simulink model "Aircraft6dof"  (R2023b)
settings: Solver=ode4  StartTime=startTime  StopTime=stopTime  FixedStep=stepTime  RelTol=1e-3  EnableMultiTasking=on
values from neighbouring files (symbols this model uses):
  a0_s2 = 0    [SetupForTrimAndLin_Aircraft6dof.m]
  a0_s3 = 0    [SetupForTrimAndLin_Aircraft6dof.m]
  a0_s4 = 0.05    [SetupForTrimAndLin_Aircraft6dof.m]
  a0_s5 = 0.05    [SetupForTrimAndLin_Aircraft6dof.m]
  AR_s2 = b_s2 / c_s2    [SetupForTrimAndLin_Aircraft6dof.m]
  AR_s3 = b_s3 / c_s3    [SetupForTrimAndLin_Aircraft6dof.m]
  AR_s4 = (b_s4+b_s5) / c_s4    [SetupForTrimAndLin_Aircraft6dof.m]
  AR_s5 = (b_s4+b_s5) / c_s5    [SetupForTrimAndLin_Aircraft6dof.m]
  ARvecP1 = ARvecUIUCp1 * 30/pi * 2    [SetupForTrimAndLin_Aircraft6dof.m]
  c_s2 = componentMassesAndGeom(3,2)    [SetupForTrimAndLin_Aircraft6dof.m]
  c_s3 = componentMassesAndGeom(4,2)    [SetupForTrimAndLin_Aircraft6dof.m]
  c_s4 = componentMassesAndGeom(1,2)    [SetupForTrimAndLin_Aircraft6dof.m]
  c_s5 = componentMassesAndGeom(2,2)    [SetupForTrimAndLin_Aircraft6dof.m]
  CD0_s2 = 0.01    [SetupForTrimAndLin_Aircraft6dof.m]
  CD0_s3 = 0.01    [SetupForTrimAndLin_Aircraft6dof.m]
  CD0_s4 = 0.01    [SetupForTrimAndLin_Aircraft6dof.m]
  CD0_s5 = 0.01    [SetupForTrimAndLin_Aircraft6dof.m]
  CDa_s2 = 1    [SetupForTrimAndLin_Aircraft6dof.m]
  CDa_s3 = 1    [SetupForTrimAndLin_Aircraft6dof.m]
  CDa_s4 = 1    [SetupForTrimAndLin_Aircraft6dof.m]
  CDa_s5 = 1    [SetupForTrimAndLin_Aircraft6dof.m]
  CL0_s2 = 0    [SetupForTrimAndLin_Aircraft6dof.m]
  CL0_s3 = 0    [SetupForTrimAndLin_Aircraft6dof.m]
  CL0_s4 = 0.05    [SetupForTrimAndLin_Aircraft6dof.m]
  CL0_s5 = 0.05    [SetupForTrimAndLin_Aircraft6dof.m]
  CM0_s2 = 0    [SetupForTrimAndLin_Aircraft6dof.m]
  CM0_s3 = 0    [SetupForTrimAndLin_Aircraft6dof.m]
  CM0_s4 = -0.05    [SetupForTrimAndLin_Aircraft6dof.m]
  CM0_s5 = -0.05    [SetupForTrimAndLin_Aircraft6dof.m]
  CMa_s2 = 0    [SetupForTrimAndLin_Aircraft6dof.m]
  CMa_s3 = 0    [SetupForTrimAndLin_Aircraft6dof.m]
  CMa_s4 = 0    [SetupForTrimAndLin_Aircraft6dof.m]
  CMa_s5 = 0    [SetupForTrimAndLin_Aircraft6dof.m]
  CQvecP1 = CPvecP1    [SetupForTrimAndLin_Aircraft6dof.m]
  CTvecP1 = CTvecUIUCp1 * 2 * (1/(2*pi))^2 * (2^4)    [SetupForTrimAndLin_Aircraft6dof.m]
  dCL_du = 3    [SetupForTrimAndLin_Aircraft6dof.m]
  dE_0 = 0    [SetupForTrimAndLin_Aircraft6dof.m]
  dEL_0 = 0    [SetupForTrimAndLin_Aircraft6dof.m]
  DeMixMatrix = inv(MixMatrix)    [SetupForTrimAndLin_Aircraft6dof.m]
  dER_0 = 0    [SetupForTrimAndLin_Aircraft6dof.m]
  dR_0 = 0    [SetupForTrimAndLin_Aircraft6dof.m]
  e_s2 = 0.8    [SetupForTrimAndLin_Aircraft6dof.m]
  e_s3 = 0.8    [SetupForTrimAndLin_Aircraft6dof.m]
  e_s4 = 0.9    [SetupForTrimAndLin_Aircraft6dof.m]
  e_s5 = 0.9    [SetupForTrimAndLin_Aircraft6dof.m]
  elevator_vector = [0  0  0.1    0.1   -0.1    -0.1  0       0  ]    [SetupAndRun_Aircraft6dof.m]
  g_E_N = [0; 0; 9.81]*1    [SetupAndRun_Aircraft6dof.m]    (also in SetupForTrimAndLin_Aircraft6dof.m = [0; 0; 9.81])
  i_s2 = -0.1    [SetupForTrimAndLin_Aircraft6dof.m]
  i_s3 = 0    [SetupForTrimAndLin_Aircraft6dof.m]
  i_s4 = 0.0    (= 0)    [SetupForTrimAndLin_Aircraft6dof.m]
  i_s5 = 0.0    (= 0)    [SetupForTrimAndLin_Aircraft6dof.m]
  InitAtt = InitAtt_deg * deg2rad    [SetupAndRun_Aircraft6dof.m]    (also in SetupForTrimAndLin_Aircraft6dof.m)
  InitPos = InitPos_deg .* [deg2rad; deg2rad; 1]    [SetupAndRun_Aircraft6dof.m]    (also in SetupForTrimAndLin_Aircraft6dof.m)
  InitRates = Rates_Trim    [SetupAndRun_Aircraft6dof.m]    (also in SetupForTrimAndLin_Aircraft6dof.m = [0; 0; 0])
  InitVel = Vel_B_BA_Trim    [SetupAndRun_Aircraft6dof.m]    (also in SetupForTrimAndLin_Aircraft6dof.m = [15; 0; 0])
  Io_motor = 1.6    [SetupForTrimAndLin_Aircraft6dof.m]
  J = zeros(3,3)    [DefineAircraftGeometry.m]    (also in InitializeModel.m = ASW.RotationalInertiaMatrix; SetupAndRun_Aircraft6dof.m = [0.049 0 -0.0004; 0 0.022 0; -0.0004 0 0.071]; SetupForTrimAndLin_Aircraft6dof.m)
  Ki_motor = 0.009549    [SetupForTrimAndLin_Aircraft6dof.m]
  m = sum(obj.componentMassesAndGeom(:,1))    [DefineAircraftGeometry.m]    (also in SetupForTrimAndLin_Aircraft6dof.m = sum(componentMassesAndGeom(:,1)))
  MixMatrix = [-1 1 0 0 ... (first row only)    [SetupForTrimAndLin_Aircraft6dof.m]
  n_p1 = [1; 0; 0]    [SetupForTrimAndLin_Aircraft6dof.m]
  n_s2 = [0; 0; -1]    [SetupForTrimAndLin_Aircraft6dof.m]
  n_s3 = [0; 1; 0]    [SetupForTrimAndLin_Aircraft6dof.m]
  n_s4 = [0; sin(0*pi/180);  -cos(0*pi/180)]    [SetupForTrimAndLin_Aircraft6dof.m]
  n_s5 = [0; sin(0*pi/180);  -cos(0*pi/180)]    [SetupForTrimAndLin_Aircraft6dof.m]
  nCellsSeries = 6    [SetupForTrimAndLin_Aircraft6dof.m]
  om_motor_init = 0    [SetupForTrimAndLin_Aircraft6dof.m]
  R_p1 = componentMassesAndGeom(11,3)/2    [SetupForTrimAndLin_Aircraft6dof.m]
  Rearth = 6371000    [SetupForTrimAndLin_Aircraft6dof.m]
  Rmotor = 0.4    [SetupForTrimAndLin_Aircraft6dof.m]
  rudder_vector = [0  0  -0.1   -0.1 0      0     0.1     0.1   0       0  ]    [SetupAndRun_Aircraft6dof.m]
  S_s2 = c_s2 * b_s2    [SetupForTrimAndLin_Aircraft6dof.m]
  S_s3 = c_s3 * b_s3    [SetupForTrimAndLin_Aircraft6dof.m]
  S_s4 = c_s4 * b_s4    [SetupForTrimAndLin_Aircraft6dof.m]
  S_s5 = c_s5 * b_s5    [SetupForTrimAndLin_Aircraft6dof.m]
  S_u_s2 = c_u_s2*b_s2    [SetupForTrimAndLin_Aircraft6dof.m]
  S_u_s3 = c_u_s3*b_s3    [SetupForTrimAndLin_Aircraft6dof.m]
  S_u_s4 = c_u_s4*b_s4    [SetupForTrimAndLin_Aircraft6dof.m]
  S_u_s5 = c_u_s5*b_s5    [SetupForTrimAndLin_Aircraft6dof.m]
  tauE = 0.1    [SetupForTrimAndLin_Aircraft6dof.m]
  tauEL = 0.1    [SetupForTrimAndLin_Aircraft6dof.m]
  tauER = 0.1    [SetupForTrimAndLin_Aircraft6dof.m]
  tauR = 0.1    [SetupForTrimAndLin_Aircraft6dof.m]
  time_vector_elevator = [0  10 10.001 100   100.001 200   200.001 10000]    [SetupAndRun_Aircraft6dof.m]
  time_vector_rudder = [0  10 10.001 70   70.001 200   200.001 300   300.001 10000]    [SetupAndRun_Aircraft6dof.m]
  v_N_AE = [0; 0; 0]    [SetupAndRun_Aircraft6dof.m]    (also in SetupForTrimAndLin_Aircraft6dof.m)
  VcellMax = 4.2    [SetupForTrimAndLin_Aircraft6dof.m]
  Vel_W_Trim = [norm(Vel_B_BA_Trim); atan2(Vel_B_BA_Trim(3),Vel_B_BA_Trim(1)); asin(Vel_B_BA_Trim(2)/norm(Vel_B_BA_Trim)) ]    [TrimAndLinearize_ATT_wInputs_Aircraft6dof.m]
  x_cm = sum(obj.componentMassesAndGeom(:,1) .* obj.componentMassesAndGeom(:,5:7)) / m    [DefineAircraftGeometry.m]    (also in SetupForTrimAndLin_Aircraft6dof.m = x_cm')
  x_p1 = componentMassesAndGeom(11,5:7)'    [SetupForTrimAndLin_Aircraft6dof.m]
  x_s2 = [componentMassesAndGeom(3,5) + (1/4)*componentMassesAndGeom(3,2); componentMassesAndGeom(3,6);componentMassesAndGeom(3,7)]    [SetupForTrimAndLin_Aircraft6dof.m]
  x_s3 = [componentMassesAndGeom(4,5) + (1/4)*componentMassesAndGeom(4,2); componentMassesAndGeom(4,6);componentMassesAndGeom(4,7)]    [SetupForTrimAndLin_Aircraft6dof.m]
  x_s4 = [componentMassesAndGeom(1,5) + (1/4)*componentMassesAndGeom(1,2); componentMassesAndGeom(1,6);componentMassesAndGeom(1,7)]    [SetupForTrimAndLin_Aircraft6dof.m]
  x_s5 = [componentMassesAndGeom(2,5) + (1/4)*componentMassesAndGeom(2,2); componentMassesAndGeom(2,6);componentMassesAndGeom(2,7)]    [SetupForTrimAndLin_Aircraft6dof.m]
undefined symbols (not defined in the file or in its folder): InitQuat, J_int, K_decouple, K_lqr, n_int, reg_lqg, X_trim, Y_trim
libraries: vrlib x8, simulink x7, aerolibfltsims x1
(part 1 of 3)
settings Model: Creator=McArthur  LastModifiedBy=prafulsigdel
settings SolverCC: AlgebraicLoopSolver=TrustRegion
settings DataIOCC: LimitDataPoints=on  SaveFormat=StructureWithTime  ReturnWorkspaceOutputs=off
settings OptimizationCC: LifeSpan=inf
settings DebuggingCC: UnconnectedInputMsg=warning  UnconnectedOutputMsg=warning  UnconnectedLineMsg=warning  SFUnexpectedBacktrackingDiag=warning  SFNoUnconditionalDefaultTransitionDiag=warning  SFExecutionAtInitializationDiag=none  ArithmeticOperatorsInVariantConditions=warning
settings HardwareCC: ProdBitPerSizeT=32  ProdBitPerPtrDiffT=32  ProdWordSize=32  ProdHWDeviceType=Specified
settings ModelReferenceCC: EnableRefExpFcnMdlSchedulingChecks=on  PropagateSignalLabelsOutOfModel=off
settings SFSimCC: SimUseLocalCustomCode=off  CustomCodeUndefinedFunction=UseInterfaceOnly
settings RTWCC: RTWUseLocalCustomCode=off
settings CodeAppCC: StateflowObjectComments=on
settings GRTTargetCC: TargetLangStandard=C89/C90 (ANSI)
settings ConfigComp: CovMetricSettings=dw  CovSaveCumulativeToWorkspaceVar=on  CovSaveSingleToWorkspaceVar=on  CovExternalEMLEnable=off

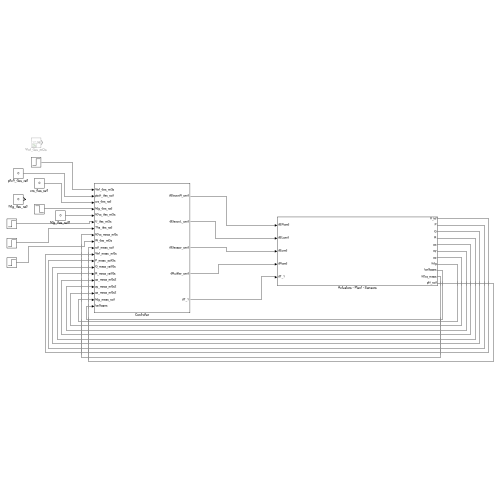
[thumbnail: Simulink's stored preview of the top-level diagram]
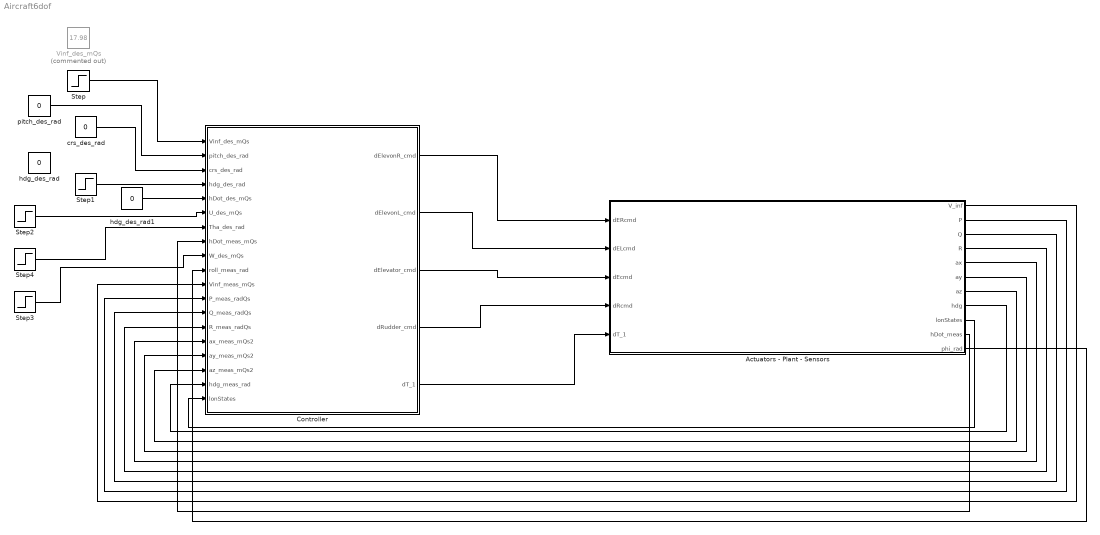
== system Aircraft6dof ==
  Actuators - Plant - Sensors : Subsystem
  Controller : Subsystem
  Step : Step  Time=9  Before=Vel_W_Trim(1)  After=Vel_W_Trim(1)+3  SampleTime=0
  Step1 : Step  Time=21  After=-170*pi/180  SampleTime=0
  Step2 : Step  Time=9  Before=X_trim(4)  After=X_trim(4)+3  SampleTime=0
  Step3 : Step  Time=9  Before=X_trim(6)  After=X_trim(6)  SampleTime=0
  Step4 : Step  Time=9  Before=X_trim(2)  After=X_trim(2)  SampleTime=0
  Vinf_des_mQs : Constant  Commented=on  Value=17.98
  crs_des_rad : Constant  Value=0
  hdg_des_rad : Constant  Value=0
  hdg_des_rad1 : Constant  Value=0
  pitch_des_rad : Constant  Value=0
  wires:
  Actuators - Plant - Sensors/1(V_inf) -> Controller/11(Vinf_meas_mQs)
  Actuators - Plant - Sensors/8(hdg) -> Controller/18(hdg_meas_rad)
  Actuators - Plant - Sensors/7(az) -> Controller/17(az_meas_mQs2)
  Actuators - Plant - Sensors/6(ay) -> Controller/16(ay_meas_mQs2)
  Actuators - Plant - Sensors/5(ax) -> Controller/15(ax_meas_mQs2)
  Actuators - Plant - Sensors/4(R) -> Controller/14(R_meas_radQs)
  Actuators - Plant - Sensors/3(Q) -> Controller/13(Q_meas_radQs)
  Actuators - Plant - Sensors/2(P) -> Controller/12(P_meas_radQs)
  Step/1 -> Controller/1(Vinf_des_mQs)
  pitch_des_rad/1 -> Controller/2(pitch_des_rad)
  crs_des_rad/1 -> Controller/3(crs_des_rad)
  Step1/1 -> Controller/4(hdg_des_rad)
  Controller/2(dElevonL_cmd) -> Actuators - Plant - Sensors/2(dELcmd)
  Controller/1(dElevonR_cmd) -> Actuators - Plant - Sensors/1(dERcmd)
  Controller/3(dElevator_cmd) -> Actuators - Plant - Sensors/3(dEcmd)
  Controller/4(dRudder_cmd) -> Actuators - Plant - Sensors/4(dRcmd)
  Actuators - Plant - Sensors/9(lonStates) -> Controller/19(lonStates)
  Step3/1 -> Controller/9(W_des_mQs)
  Step4/1 -> Controller/7(Tha_des_rad)
  Step2/1 -> Controller/6(U_des_mQs)
  Controller/5(dT_1) -> Actuators - Plant - Sensors/5(dT_1)
  hdg_des_rad1/1 -> Controller/5(hDot_des_mQs)
  Actuators - Plant - Sensors/10(hDot_meas) -> Controller/8(hDot_meas_mQs)
  Actuators - Plant - Sensors/11(phi_rad) -> Controller/10(roll_meas_rad)

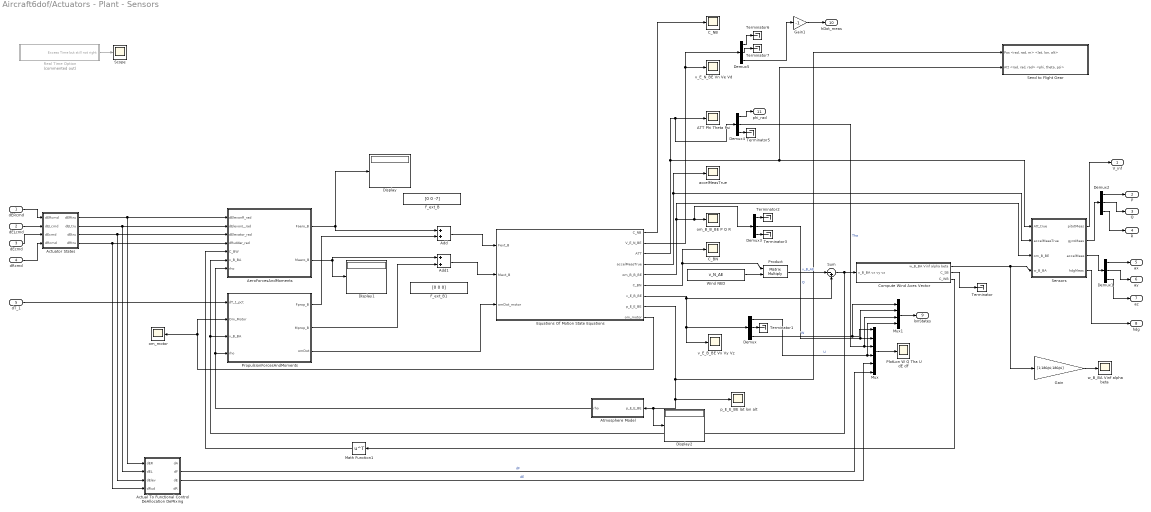
== system Aircraft6dof/Actuators - Plant - Sensors ==
  dERcmd : Inport
  dELcmd : Inport  Port=2
  dEcmd : Inport  Port=3
  dRcmd : Inport  Port=4
  dT_1 : Inport  Port=5
  ATT Phi Theta Psi : Scope
  Actual To Functional Control DeAllocation DeMixing : Subsystem
  Actuator States : Subsystem
  Add : Sum
  Add1 : Sum
  AeroForcesAndMoments : Subsystem
  Atmosphere Model : Subsystem
  C_BN : Scope
  C_NB : Scope
  Compute Wind Axes Vector : Subsystem
  Demux{,1..5} (6 alike) : Demux  Outputs=3
  Display : Display
  Display1 : Display
  Display2 : Display
  Equations Of Motion State Equations : Subsystem
  F_ext_B : Constant  Value=[0 0 -7]
  F_ext_B1 : Constant  Value=[0 0 0]
  Gain : Gain  Gain=[1;180/pi;180/pi]
  Gain1 : Gain  Gain=-1
  Math Function1 : Math  Operator=transpose  SignedPower=on
  Mux : Mux  Inputs=6
  Mux1 : Mux
  PlotLon W Q Tha U dE dF : Scope
  Product : Product  Multiplication=Matrix(*)
  PropulsionForcesAndMoments : Subsystem
  Real Time Option : Subsystem  Commented=on
  Scope : Scope
  Send to Flight Gear : Subsystem
  Sensors : Subsystem
  Sum : Sum  Inputs=|-+
  Terminator{,1..3,5..7} (7 alike) : Terminator
  Wind NED : Constant  Value=v_N_AE
  accelMeasTrue : Scope
  om_B_B_BE P Q R : Scope
  om_motor : Scope
  p_E_E_BE lat lon alt : Scope
  v_E_B_BE Vx Vy Vz : Scope
  v_E_N_BE Vn Ve Vd : Scope
  w_B_BA Vinf alpha beta : Scope
  V_inf : Outport  VectorParamsAs1DForOutWhenUnconnected=off
  P : Outport  Port=2  VectorParamsAs1DForOutWhenUnconnected=off
  Q : Outport  Port=3  VectorParamsAs1DForOutWhenUnconnected=off
  R : Outport  Port=4  VectorParamsAs1DForOutWhenUnconnected=off
  ax : Outport  Port=5  VectorParamsAs1DForOutWhenUnconnected=off
  ay : Outport  Port=6  VectorParamsAs1DForOutWhenUnconnected=off
  az : Outport  Port=7  VectorParamsAs1DForOutWhenUnconnected=off
  hdg : Outport  Port=8  VectorParamsAs1DForOutWhenUnconnected=off
  lonStates : Outport  Port=9  VectorParamsAs1DForOutWhenUnconnected=off
  hDot_meas : Outport  Port=10  VectorParamsAs1DForOutWhenUnconnected=off
  phi_rad : Outport  Port=11  VectorParamsAs1DForOutWhenUnconnected=off
  wires:
  Real Time Option/1(Excess Time but still not right) -> Scope/1
  AeroForcesAndMoments/2(Maero_B) -> Add1/1, Display1/1
  PropulsionForcesAndMoments/3(omDot) -> Equations Of Motion State Equations/3(omDot_motor)
  AeroForcesAndMoments/1(Faero_B) -> Add/1, Display/1
  Equations Of Motion State Equations/8(p_E_E_BE) -> Send to Flight Gear/1("Pos <rad, rad, m> <lat, lon, alt>"), Display2/1, Atmosphere Model/1(p_E_E_BE), p_E_E_BE lat lon alt/1
  Equations Of Motion State Equations/2(V_E_N_BE) -> Demux5/1, v_E_N_BE Vn Ve Vd/1
  Equations Of Motion State Equations/1(C_NB) -> C_NB/1
  Sum/1 -> PropulsionForcesAndMoments/3(v_B_BA), AeroForcesAndMoments/6(v_B_BA), Compute Wind Axes Vector/1(v_B_BA vx vy vz)
  Compute Wind Axes Vector/3(C_WB) -> Math Function1/1
  Math Function1/1 -> AeroForcesAndMoments/5(C_BW)
  Equations Of Motion State Equations/5(om_B_B_BE) -> Sensors/3(om_B_BE), Demux3/1, om_B_B_BE P Q R/1
  Equations Of Motion State Equations/6(C_BN) -> C_BN/1, Product/1
  Demux2/2 -> Q/1
  Demux2/3 -> R/1
  Demux2/1 -> P/1
  Product/1 -> Sum/1  "v_B_AE"
  Gain/1 -> w_B_BA Vinf alpha beta/1
  Atmosphere Model/1(rho) -> PropulsionForcesAndMoments/4(rho), AeroForcesAndMoments/7(rho)
  Compute Wind Axes Vector/1(w_B_BA Vinf alpha beta) -> Gain/1, Sensors/4(w_B_BA)
  Compute Wind Axes Vector/2(C_SB) -> Terminator/1
  Equations Of Motion State Equations/7(v_E_B_BE) -> Sum/2, v_E_B_BE Vx Vy Vz/1, Demux/1
  Sensors/1(pitotMeas) -> V_inf/1
  Sensors/2(gyroMeas) -> Demux2/1
  Equations Of Motion State Equations/4(accelMeasTrue) -> Sensors/2(accelMeasTrue), accelMeasTrue/1
  Wind NED/1 -> Product/2
  Demux1/1 -> ax/1
  Demux1/2 -> ay/1
  Demux1/3 -> az/1
  Sensors/3(accelMeas) -> Demux1/1
  Sensors/4(hdgMeas) -> hdg/1
  Actuator States/4(dRtru) -> Actual To Functional Control DeAllocation DeMixing/4(dRud), AeroForcesAndMoments/4(dRudder_rad)
  Actuator States/3(dEtru) -> Actual To Functional Control DeAllocation DeMixing/3(dElev), AeroForcesAndMoments/3(dElevator_rad)
  Actuator States/2(dELtru) -> Actual To Functional Control DeAllocation DeMixing/2(dEL), AeroForcesAndMoments/2(dElevonL_rad)
  Actuator States/1(dERtru) -> Actual To Functional Control DeAllocation DeMixing/1(dER), AeroForcesAndMoments/1(dElevonR_rad)
  dERcmd/1 -> Actuator States/1(dERcmd)
  dELcmd/1 -> Actuator States/2(dELcmd)
  dEcmd/1 -> Actuator States/3(dEcmd)
  dRcmd/1 -> Actuator States/4(dRcmd)
  Mux/1 -> PlotLon W Q Tha U dE dF/1
  Demux/3 -> Mux1/1, Mux/1  "W"
  Demux/1 -> Mux1/4, Mux/4  "U"
  Demux/2 -> Terminator1/1
  Demux3/2 -> Mux1/2, Mux/2  "Q"
  Demux3/1 -> Terminator2/1
  Demux3/3 -> Terminator3/1
  Equations Of Motion State Equations/3(ATT) -> Demux4/1, ATT Phi Theta Psi/1, Send to Flight Gear/2("Att <rad, rad, rad> <phi, theta, psi>"), Sensors/1(Att_true)
  Demux4/2 -> Mux1/3, Mux/3  "Tha"
  Demux4/1 -> phi_rad/1
  Demux4/3 -> Terminator5/1
  Actual To Functional Control DeAllocation DeMixing/3(dE) -> Mux/5  "dE"
  Actual To Functional Control DeAllocation DeMixing/2(dF) -> Mux/6  "dF"
  Mux1/1 -> lonStates/1
  Add/1 -> Equations Of Motion State Equations/1(Fext_B)
  Add1/1 -> Equations Of Motion State Equations/2(Mext_B)
  dT_1/1 -> PropulsionForcesAndMoments/1(dT_1_pct)
  Equations Of Motion State Equations/9(om_motor) -> PropulsionForcesAndMoments/2(Om_Motor), om_motor/1
  PropulsionForcesAndMoments/1(Fprop_B) -> Add/2
  PropulsionForcesAndMoments/2(Mprop_B) -> Add1/2
  Demux5/3 -> Gain1/1
  Gain1/1 -> hDot_meas/1
  Demux5/1 -> Terminator6/1
  Demux5/2 -> Terminator7/1

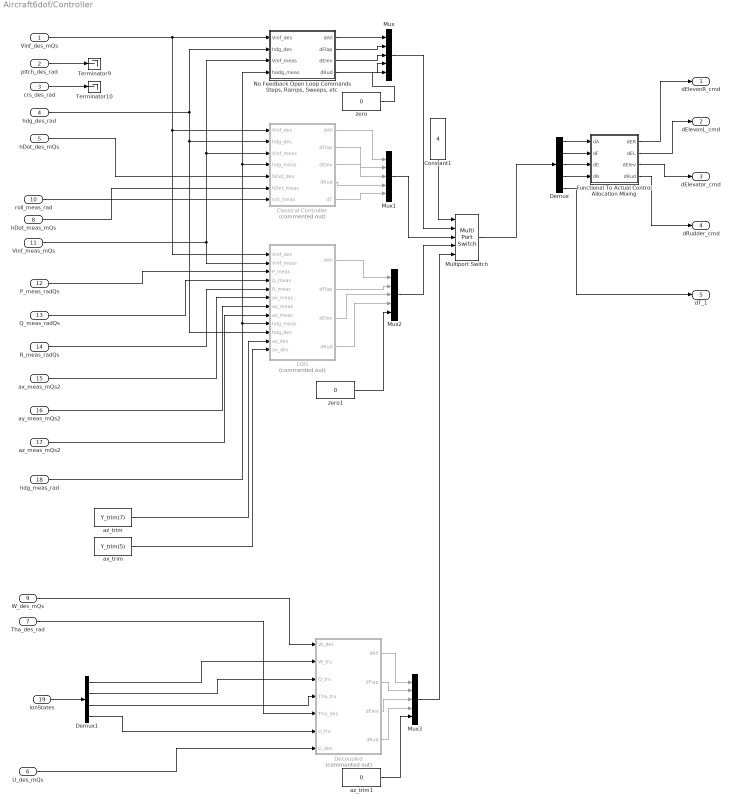
== system Aircraft6dof/Controller ==
  Vinf_des_mQs : Inport
  pitch_des_rad : Inport  Port=2
  crs_des_rad : Inport  Port=3
  hdg_des_rad : Inport  Port=4
  hDot_des_mQs : Inport  Port=5
  U_des_mQs : Inport  Port=6
  Tha_des_rad : Inport  Port=7
  hDot_meas_mQs : Inport  Port=8
  W_des_mQs : Inport  Port=9
  roll_meas_rad : Inport  Port=10
  Vinf_meas_mQs : Inport  Port=11
  P_meas_radQs : Inport  Port=12
  Q_meas_radQs : Inport  Port=13
  R_meas_radQs : Inport  Port=14
  ax_meas_mQs2 : Inport  Port=15
  ay_meas_mQs2 : Inport  Port=16
  az_meas_mQs2 : Inport  Port=17
  hdg_meas_rad : Inport  Port=18
  lonStates : Inport  Port=19
  Classical Controller : Subsystem  Commented=on
  Constant1 : Constant  Value=4
  Decoupled : Subsystem  Commented=on
  Demux : Demux  Outputs=5
  Demux1 : Demux
  Functional To Actual Control Allocation Mixing : Subsystem
  LQG : Subsystem  Commented=on
  Multiport Switch : MultiPortSwitch  Inputs=4  SaturateOnIntegerOverflow=off  InputSameDT=off
  Mux{,1..3} (4 alike) : Mux  Inputs=5
  "No Feedback Open Loop Commands Steps, Ramps, Sweeps, etc" : Subsystem
  Terminator10 : Terminator
  Terminator9 : Terminator
  ax_trim : Constant  Value=Y_trim(5)
  az_trim : Constant  Value=Y_trim(7)
  az_trim1 : Constant  Value=0
  zero : Constant  Value=0
  zero1 : Constant  Value=0
  dElevonR_cmd : Outport  VectorParamsAs1DForOutWhenUnconnected=off
  dElevonL_cmd : Outport  Port=2  VectorParamsAs1DForOutWhenUnconnected=off
  dElevator_cmd : Outport  Port=3  VectorParamsAs1DForOutWhenUnconnected=off
  dRudder_cmd : Outport  Port=4  VectorParamsAs1DForOutWhenUnconnected=off
  dT_1 : Outport  Port=5  VectorParamsAs1DForOutWhenUnconnected=off
  wires:
  P_meas_radQs/1 -> LQG/3(P_meas)
  Q_meas_radQs/1 -> LQG/4(Q_meas)
  ay_meas_mQs2/1 -> LQG/7(ay_meas)
  ax_meas_mQs2/1 -> LQG/6(ax_meas)
  R_meas_radQs/1 -> LQG/5(R_meas)
  az_meas_mQs2/1 -> LQG/8(az_meas)
  crs_des_rad/1 -> Terminator10/1
  pitch_des_rad/1 -> Terminator9/1
  Functional To Actual Control Allocation Mixing/1(dER) -> dElevonR_cmd/1
  Functional To Actual Control Allocation Mixing/2(dEL) -> dElevonL_cmd/1
  Functional To Actual Control Allocation Mixing/3(dElev) -> dElevator_cmd/1
  Functional To Actual Control Allocation Mixing/4(dRud) -> dRudder_cmd/1
  hdg_des_rad/1 -> LQG/10(hdg_des), Classical Controller/2(hdg_des), "No Feedback Open Loop Commands Steps, Ramps, Sweeps, etc"/2(hdg_des)
  Vinf_meas_mQs/1 -> LQG/2(Vinf_meas), "No Feedback Open Loop Commands Steps, Ramps, Sweeps, etc"/3(Vinf_meas), Classical Controller/3(Vinf_meas)
  hdg_meas_rad/1 -> Classical Controller/4(hdg_meas), "No Feedback Open Loop Commands Steps, Ramps, Sweeps, etc"/4(hadg_meas), LQG/9(hdg_meas)
  "No Feedback Open Loop Commands Steps, Ramps, Sweeps, etc"/1(dAil) -> Mux/1
  "No Feedback Open Loop Commands Steps, Ramps, Sweeps, etc"/2(dFlap) -> Mux/2
  "No Feedback Open Loop Commands Steps, Ramps, Sweeps, etc"/3(dElev) -> Mux/3
  "No Feedback Open Loop Commands Steps, Ramps, Sweeps, etc"/4(dRud) -> Mux/4
  Mux/1 -> Multiport Switch/2
  Constant1/1 -> Multiport Switch/1
  Classical Controller/1(dAil) -> Mux1/1
  Classical Controller/4(dRud) -> Mux1/4
  Classical Controller/3(dElev) -> Mux1/3
  Classical Controller/2(dFlap) -> Mux1/2
  Mux1/1 -> Multiport Switch/3
  Demux/3 -> Functional To Actual Control Allocation Mixing/3(dE)
  Demux/2 -> Functional To Actual Control Allocation Mixing/2(dF)
  Demux/1 -> Functional To Actual Control Allocation Mixing/1(dA)
  Demux/4 -> Functional To Actual Control Allocation Mixing/4(dR)
  Multiport Switch/1 -> Demux/1
  LQG/1(dAil) -> Mux2/1
  LQG/4(dRud) -> Mux2/4
  LQG/3(dElev) -> Mux2/3
  LQG/2(dFlap) -> Mux2/2
  Mux2/1 -> Multiport Switch/4
  Vinf_des_mQs/1 -> "No Feedback Open Loop Commands Steps, Ramps, Sweeps, etc"/1(Vinf_des), LQG/1(Vinf_des), Classical Controller/1(Vinf_des)
  az_trim/1 -> LQG/11(az_des)
  ax_trim/1 -> LQG/12(ax_des)
  Decoupled/1(dAil) -> Mux3/1
  Decoupled/2(dFlap) -> Mux3/2
  Decoupled/3(dElev) -> Mux3/3
  Decoupled/4(dRud) -> Mux3/4
  Mux3/1 -> Multiport Switch/5
  lonStates/1 -> Demux1/1
  Demux1/1 -> Decoupled/2(W_tru)
  Demux1/2 -> Decoupled/3(Q_tru)
  Demux1/3 -> Decoupled/4(Tha_tru)
  Demux1/4 -> Decoupled/6(U_tru)
  W_des_mQs/1 -> Decoupled/1(W_des)
  Tha_des_rad/1 -> Decoupled/5(Tha_des)
  U_des_mQs/1 -> Decoupled/7(U_des)
  Demux/5 -> dT_1/1
  hDot_des_mQs/1 -> Classical Controller/5(hDot_des)
  hDot_meas_mQs/1 -> Classical Controller/6(hDot_meas)
  roll_meas_rad/1 -> Classical Controller/7(roll_meas)
  Classical Controller/5(dT) -> Mux1/5
  zero/1 -> Mux/5
  zero1/1 -> Mux2/5
  az_trim1/1 -> Mux3/5

== system Aircraft6dof/Actuators - Plant - Sensors/Actual To Functional Control DeAllocation DeMixing ==
  dER : Inport
  dEL : Inport  Port=2
  dElev : Inport  Port=3
  dRud : Inport  Port=4
  Constant1 : Constant  Value=DeMixMatrix
  Demux : Demux
  Mux : Mux
  Product1 : Product  Multiplication=Matrix(*)
  dA : Outport  VectorParamsAs1DForOutWhenUnconnected=off
  dF : Outport  Port=2  VectorParamsAs1DForOutWhenUnconnected=off
  dE : Outport  Port=3  VectorParamsAs1DForOutWhenUnconnected=off
  dR : Outport  Port=4  VectorParamsAs1DForOutWhenUnconnected=off
  wires:
  dER/1 -> Mux/1
  dEL/1 -> Mux/2
  dElev/1 -> Mux/3
  dRud/1 -> Mux/4
  Demux/2 -> dF/1
  Constant1/1 -> Product1/1
  Mux/1 -> Product1/2
  Demux/1 -> dA/1
  Demux/4 -> dR/1
  Demux/3 -> dE/1
  Product1/1 -> Demux/1

== system Aircraft6dof/Actuators - Plant - Sensors/Actuator States ==
  dERcmd : Inport
  dELcmd : Inport  Port=2
  dEcmd : Inport  Port=3
  dRcmd : Inport  Port=4
  Constant : Constant  Value=dER_0
  Constant1 : Constant  Value=dEL_0
  Constant2 : Constant  Value=dE_0
  Constant3 : Constant  Value=dR_0
  Gain : Gain  Gain=1/tauER
  Gain1 : Gain  Gain=1/tauEL
  Gain2 : Gain  Gain=1/tauE
  Gain3 : Gain  Gain=1/tauR
  Sum{,1..3} (4 alike) : Sum  Inputs=|+-
  dE : Integrator  InitialConditionSource=external
  dEL : Integrator  InitialConditionSource=external
  dER : Integrator  InitialConditionSource=external
  dR : Integrator  InitialConditionSource=external
  dERtru : Outport  VectorParamsAs1DForOutWhenUnconnected=off
  dELtru : Outport  Port=2  VectorParamsAs1DForOutWhenUnconnected=off
  dEtru : Outport  Port=3  VectorParamsAs1DForOutWhenUnconnected=off
  dRtru : Outport  Port=4  VectorParamsAs1DForOutWhenUnconnected=off
  wires:
  dER/1 -> Sum/2, dERtru/1
  dERcmd/1 -> Sum/1
  Gain/1 -> dER/1
  Sum/1 -> Gain/1
  Constant/1 -> dER/2
  dEL/1 -> Sum1/2, dELtru/1
  dELcmd/1 -> Sum1/1
  Gain1/1 -> dEL/1
  Sum1/1 -> Gain1/1
  Constant1/1 -> dEL/2
  dE/1 -> Sum2/2, dEtru/1
  dEcmd/1 -> Sum2/1
  Gain2/1 -> dE/1
  Sum2/1 -> Gain2/1
  Constant2/1 -> dE/2
  dR/1 -> Sum3/2, dRtru/1
  dRcmd/1 -> Sum3/1
  Gain3/1 -> dR/1
  Sum3/1 -> Gain3/1
  Constant3/1 -> dR/2

== system Aircraft6dof/Actuators - Plant - Sensors/AeroForcesAndMoments ==
  dElevonR_rad : Inport
  dElevonL_rad : Inport  Port=2
  dElevator_rad : Inport  Port=3
  dRudder_rad : Inport  Port=4
  C_BW : Inport  Port=5
  v_B_BA : Inport  Port=6
  rho : Inport  Port=7
  Add : Sum  Inputs=++++
  Add1 : Sum  Inputs=++++
  Display1 : Display
  Display3 : Display
  Surface2 : Subsystem
  Surface3 : Subsystem
  Surface4 : Subsystem
  Surface5 : Subsystem
  Faero_B : Outport  VectorParamsAs1DForOutWhenUnconnected=off
  Maero_B : Outport  Port=2  VectorParamsAs1DForOutWhenUnconnected=off
  wires:
  C_BW/1 -> Surface2/1(C_BW), Surface3/1(C_BW), Surface5/1(C_BW), Surface4/1(C_BW)
  v_B_BA/1 -> Surface3/2(v_B_BA), Surface2/2(v_B_BA), Surface5/2(v_B_BA), Surface4/2(v_B_BA)
  rho/1 -> Surface3/3(rho), Surface2/3(rho), Surface5/3(rho), Surface4/3(rho)
  Surface4/1(Fs4_B) -> Add/1
  Surface5/1(Fs5_B) -> Add/2
  Surface4/2(Ms4_B) -> Add1/1
  Surface5/2(Ms5_B) -> Add1/2
  Surface2/1(Fs2_B) -> Add/3
  Surface2/2(Ms2_B) -> Add1/3
  Add1/1 -> Display1/1, Maero_B/1
  Add/1 -> Display3/1, Faero_B/1
  Surface3/1(Fs2_B) -> Add/4
  Surface3/2(Ms2_B) -> Add1/4
  dElevonR_rad/1 -> Surface4/4(u_s#_rad)
  dElevonL_rad/1 -> Surface5/4(u_s#_rad)
  dElevator_rad/1 -> Surface2/4(u_s#_rad)
  dRudder_rad/1 -> Surface3/4(u_s#_rad)

== system Aircraft6dof/Actuators - Plant - Sensors/Atmosphere Model ==
  p_E_E_BE : Inport
  Compare To Constant : simulink/Logic and Bit Operations/Compare To Constant  relop=<=  const=11000  OutDataTypeStr=boolean
  Demux : Demux  Outputs=3
  Enhance Me Please! : Constant  Value=0
  Standard Atmosphere - Troposphere : MATLAB Function  TreatAsAtomicUnit=on
  Switch : Switch  Criteria=u2 ~= 0  Threshold=11000  SaturateOnIntegerOverflow=off  InputSameDT=off
  Terminator : Terminator
  Terminator1 : Terminator
  rho : Outport  VectorParamsAs1DForOutWhenUnconnected=off
  wires:
  p_E_E_BE/1 -> Demux/1
  Demux/1 -> Terminator/1
  Demux/2 -> Terminator1/1
  Demux/3 -> Standard Atmosphere - Troposphere/1(h), Compare To Constant/1
  Compare To Constant/1 -> Switch/2
  Standard Atmosphere - Troposphere/1(rho) -> Switch/1
  Switch/1 -> rho/1
  Enhance Me Please!/1 -> Switch/3

== system Aircraft6dof/Actuators - Plant - Sensors/Compute Wind Axes Vector ==
  v_B_BA vx vy vz : Inport
  Compute Wind DCMs : MATLAB Function  TreatAsAtomicUnit=on
  Constant : Constant  Value=[0;0;0]
  Constant1 : Constant  Value=0.001
  Demux : Demux  Outputs=3
  Display : Display
  Divide : Product  Inputs=*/
  Dot Product : DotProduct  OutDataTypeStr=Inherit: Inherit via internal rule
  MinMax : MinMax  Function=max  Inputs=2
  Mux : Mux  Inputs=3
  Saturation : Saturate  UpperLimit=1  LowerLimit=-1
  Sqrt : Sqrt
  Switch : Switch  Criteria=u2 > Threshold  SaturateOnIntegerOverflow=off  InputSameDT=off
  Trigonometric Function : Trigonometry  Operator=atan2
  Trigonometric Function1 : Trigonometry  Operator=asin
  w_B_BA Vinf alpha beta : Outport  VectorParamsAs1DForOutWhenUnconnected=off
  C_SB : Outport  Port=2  VectorParamsAs1DForOutWhenUnconnected=off
  C_WB : Outport  Port=3  VectorParamsAs1DForOutWhenUnconnected=off
  wires:
  Dot Product/1 -> Sqrt/1
  Mux/1 -> Switch/1
  Constant/1 -> Switch/3
  Trigonometric Function/1 -> Display/1, Compute Wind DCMs/2(alpha), Mux/2
  Switch/1 -> w_B_BA Vinf alpha beta/1
  Demux/3 -> Trigonometric Function/1
  v_B_BA vx vy vz/1 -> Demux/1, Dot Product/2, Dot Product/1
  Demux/1 -> Trigonometric Function/2
  Constant1/1 -> MinMax/1
  MinMax/1 -> Divide/2
  Demux/2 -> Divide/1
  Divide/1 -> Saturation/1
  Saturation/1 -> Trigonometric Function1/1
  Trigonometric Function1/1 -> Compute Wind DCMs/3(beta), Mux/3
  Sqrt/1 -> Compute Wind DCMs/1(Vinf), Mux/1, Switch/2, MinMax/2
  Compute Wind DCMs/2(C_WB) -> C_WB/1
  Compute Wind DCMs/1(C_SB) -> C_SB/1

== system Aircraft6dof/Actuators - Plant - Sensors/Equations Of Motion State Equations ==
  Fext_B : Inport
  Mext_B : Inport  Port=2
  omDot_motor : Inport  Port=3
  Earth Model : Subsystem
  MATLAB Function : MATLAB Function  Commented=on  TreatAsAtomicUnit=on
  Math Function : Math  Operator=transpose  SignedPower=on
  Product1 : Product  Multiplication=Matrix(*)
  Product2 : Product  Multiplication=Matrix(*)
  QUAT2ATT : Subsystem
  QUAT2DCM : Subsystem
  Rot Dyn (Moments) : Subsystem
  Rot Kin (Orientation) Euler : Subsystem  Commented=on
  Rot Kin (Orientation) Quaternion : Subsystem
  Trans Dyn (Forces) : Subsystem
  Trans Kin (Spherical) : Subsystem
  C_NB : Outport  VectorParamsAs1DForOutWhenUnconnected=off
  V_E_N_BE : Outport  Port=2  VectorParamsAs1DForOutWhenUnconnected=off
  ATT : Outport  Port=3  VectorParamsAs1DForOutWhenUnconnected=off
  accelMeasTrue : Outport  Port=4  VectorParamsAs1DForOutWhenUnconnected=off
  om_B_B_BE : Outport  Port=5  VectorParamsAs1DForOutWhenUnconnected=off
  C_BN : Outport  Port=6  VectorParamsAs1DForOutWhenUnconnected=off
  v_E_B_BE : Outport  Port=7  VectorParamsAs1DForOutWhenUnconnected=off
  p_E_E_BE : Outport  Port=8  VectorParamsAs1DForOutWhenUnconnected=off
  om_motor : Outport  Port=9  VectorParamsAs1DForOutWhenUnconnected=off
  wires:
  omDot_motor/1 -> Rot Dyn (Moments)/2(omDot_motor)
  Rot Dyn (Moments)/1(om_B_B_BE) -> Trans Dyn (Forces)/3(om_B_B_BE), Rot Kin (Orientation) Quaternion/1(om_B_B_BN), Rot Kin (Orientation) Euler/1(om_B_B_BN), om_B_B_BE/1
  Trans Dyn (Forces)/1(xDot_E_B_BE) -> Trans Kin (Spherical)/1(v_E_B_BE), v_E_B_BE/1, Product1/2
  Rot Kin (Orientation) Quaternion/1(q_BN) -> QUAT2DCM/1(Quat), QUAT2ATT/1(q)
  QUAT2DCM/1(DCM) -> C_BN/1, Math Function/1, Product2/1  "C_BN"
  Mext_B/1 -> Rot Dyn (Moments)/1(Mext_B)
  Fext_B/1 -> Trans Dyn (Forces)/1(Fext_B)
  QUAT2ATT/1(ATT) -> MATLAB Function/1(ATT), ATT/1
  Trans Kin (Spherical)/1(p_E_E_BE) -> Earth Model/1(p_E_E_BE), p_E_E_BE/1
  Math Function/1 -> C_NB/1, Trans Kin (Spherical)/2(C_NB), Product1/1  "C_NB"
  Product1/1 -> V_E_N_BE/1
  Earth Model/2(g_N) -> Product2/2
  Product2/1 -> Trans Dyn (Forces)/2(g_B)
  Rot Dyn (Moments)/2(om_motor) -> om_motor/1
  Trans Dyn (Forces)/2(accelMeasCG) -> accelMeasTrue/1
  Earth Model/1(Rearth) -> Trans Kin (Spherical)/3(Rearth)

== system Aircraft6dof/Actuators - Plant - Sensors/PropulsionForcesAndMoments ==
  dT_1_pct : Inport
  Om_Motor : Inport  Port=2
  v_B_BA : Inport  Port=3
  rho : Inport  Port=4
  Add : Sum  Inputs=++++
  Add1 : Sum  Inputs=++++
  Constant : Constant  Value=0
  Display1 : Display
  Display3 : Display
  PropulsionSystem1 : Subsystem
  Fprop_B : Outport  VectorParamsAs1DForOutWhenUnconnected=off
  Mprop_B : Outport  Port=2  VectorParamsAs1DForOutWhenUnconnected=off
  omDot : Outport  Port=3  VectorParamsAs1DForOutWhenUnconnected=off
  wires:
  dT_1_pct/1 -> PropulsionSystem1/4(u_p#_pct)
  Add/1 -> Fprop_B/1, Display3/1
  Add1/1 -> Mprop_B/1, Display1/1
  Constant/1 -> Add1/4, Add1/3, Add1/2, Add/4, Add/3, Add/2
  PropulsionSystem1/1(Fs4_B) -> Add/1
  rho/1 -> PropulsionSystem1/3(rho)
  v_B_BA/1 -> PropulsionSystem1/2(v_B_BA)
  Om_Motor/1 -> PropulsionSystem1/1(Om_p1)
  PropulsionSystem1/2(Ms4_B) -> Add1/1
  PropulsionSystem1/3(omDot) -> omDot/1

== system Aircraft6dof/Actuators - Plant - Sensors/Real Time Option ==
  S-Function : S-Function  FunctionName=sfun_RealTimeOption  Parameters=RatioToRealTime  SFunctionDeploymentMode=off  EnableBusSupport=off
  Timer for Real-Time : S-Function  FunctionName=sfun_RealTimeOptional  Parameters=RatioToRealTime  SFunctionDeploymentMode=off  EnableBusSupport=off
  Excess Time but still not right : Outport  VectorParamsAs1DForOutWhenUnconnected=off
  wires:
  Timer for Real-Time/1 -> Excess Time but still not right/1

== system Aircraft6dof/Actuators - Plant - Sensors/Send to Flight Gear ==
  "Pos <rad, rad, m> <lat, lon, alt>" : Inport
  "Att <rad, rad, rad> <phi, theta, psi>" : Inport  Port=2
  FlightGear Preconfigured 6DoF Animation : aerolibfltsims/FlightGear Preconfigured 6DoF Animation  xFlightGearVersion=v2019.1  DestinationIpAddress=127.0.0.1  DestinationPort=5502  SampleTime=1/10  packetVersion=24
  Mux : Mux  Inputs=2
  wires:
  "Pos <rad, rad, m> <lat, lon, alt>"/1 -> Mux/1
  "Att <rad, rad, rad> <phi, theta, psi>"/1 -> Mux/2
  Mux/1 -> FlightGear Preconfigured 6DoF Animation/1

== system Aircraft6dof/Actuators - Plant - Sensors/Sensors ==
  Att_true : Inport
  accelMeasTrue : Inport  Port=2
  om_B_BE : Inport  Port=3
  w_B_BA : Inport  Port=4
  Demux : Demux  Outputs=3
  Demux1 : Demux  Outputs=3
  Terminator{1..4} (4 alike) : Terminator
  pitotMeas : Outport  VectorParamsAs1DForOutWhenUnconnected=off
  gyroMeas : Outport  Port=2  VectorParamsAs1DForOutWhenUnconnected=off
  accelMeas : Outport  Port=3  VectorParamsAs1DForOutWhenUnconnected=off
  hdgMeas : Outport  Port=4  VectorParamsAs1DForOutWhenUnconnected=off
  wires:
  om_B_BE/1 -> gyroMeas/1
  w_B_BA/1 -> Demux/1
  Demux/3 -> Terminator1/1
  Demux/2 -> Terminator2/1
  Demux/1 -> pitotMeas/1
  accelMeasTrue/1 -> accelMeas/1
  Att_true/1 -> Demux1/1
  Demux1/1 -> Terminator3/1
  Demux1/2 -> Terminator4/1
  Demux1/3 -> hdgMeas/1

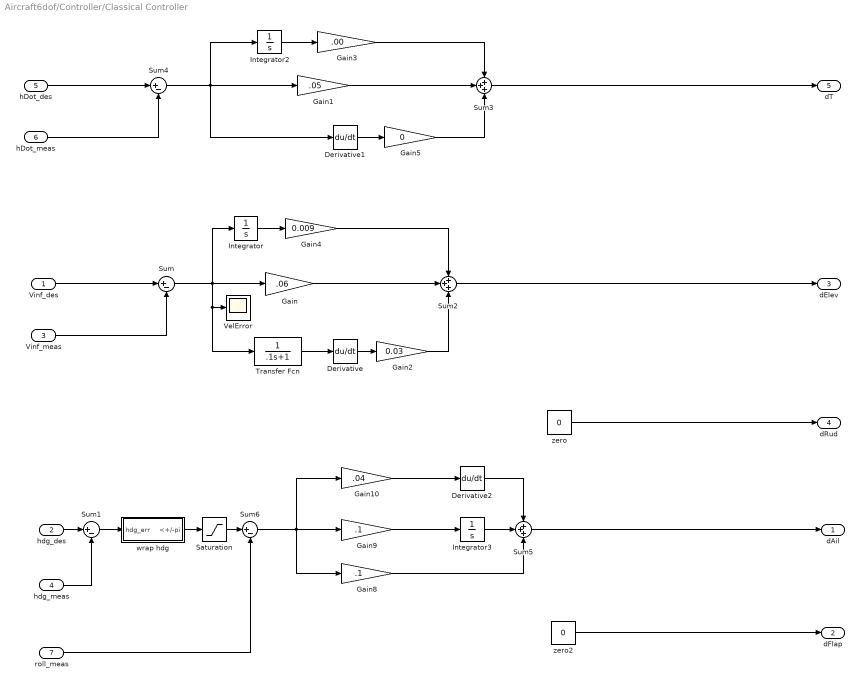
== system Aircraft6dof/Controller/Classical Controller ==
  Vinf_des : Inport
  hdg_des : Inport  Port=2
  Vinf_meas : Inport  Port=3
  hdg_meas : Inport  Port=4
  hDot_des : Inport  Port=5
  hDot_meas : Inport  Port=6
  roll_meas : Inport  Port=7
  Derivative : Derivative
  Derivative1 : Derivative
  Derivative2 : Derivative
  Gain : Gain  Gain=.06
  Gain1 : Gain  Gain=.05
  Gain10 : Gain  Gain=.04
  Gain2 : Gain  Gain=0.03
  Gain3 : Gain  Gain=.00
  Gain4 : Gain  Gain=0.009
  Gain5 : Gain  Gain=0
  Gain8 : Gain  Gain=.1
  Gain9 : Gain  Gain=.1
  Integrator : Integrator
  Integrator2 : Integrator
  Integrator3 : Integrator
  Saturation : Saturate  UpperLimit=0.3  LowerLimit=-0.3
  Sum{,1,4,6} (4 alike) : Sum  Inputs=|+-
  Sum2 : Sum  Inputs=+++
  Sum3 : Sum  Inputs=+++
  Sum5 : Sum  Inputs=+++
  Transfer Fcn : TransferFcn  Denominator=[.1 1]
  VelError : Scope
  wrap hdg : Subsystem
  zero : Constant  Value=0
  zero2 : Constant  Value=0
  dAil : Outport  VectorParamsAs1DForOutWhenUnconnected=off
  dFlap : Outport  Port=2  VectorParamsAs1DForOutWhenUnconnected=off
  dElev : Outport  Port=3  VectorParamsAs1DForOutWhenUnconnected=off
  dRud : Outport  Port=4  VectorParamsAs1DForOutWhenUnconnected=off
  dT : Outport  Port=5  VectorParamsAs1DForOutWhenUnconnected=off
  wires:
  zero2/1 -> dFlap/1
  zero/1 -> dRud/1
  Gain/1 -> Sum2/2
  Vinf_des/1 -> Sum/1
  Sum/1 -> Integrator/1, Transfer Fcn/1, VelError/1, Gain/1
  hdg_des/1 -> Sum1/1
  Sum2/1 -> dElev/1
  Integrator/1 -> Gain4/1
  Gain4/1 -> Sum2/1
  Derivative/1 -> Gain2/1
  Gain2/1 -> Sum2/3
  Vinf_meas/1 -> Sum/2
  Sum1/1 -> wrap hdg/1(hdg_err)
  Transfer Fcn/1 -> Derivative/1
  hdg_meas/1 -> Sum1/2
  hDot_des/1 -> Sum4/1
  hDot_meas/1 -> Sum4/2
  Sum4/1 -> Derivative1/1, Gain1/1, Integrator2/1
  Integrator2/1 -> Gain3/1
  Gain3/1 -> Sum3/1
  Sum6/1 -> Gain8/1, Gain10/1, Gain9/1
  Gain8/1 -> Sum5/3
  Gain9/1 -> Integrator3/1
  Integrator3/1 -> Sum5/2
  Sum5/1 -> dAil/1
  Gain10/1 -> Derivative2/1
  Derivative2/1 -> Sum5/1
  roll_meas/1 -> Sum6/2
  Saturation/1 -> Sum6/1
  wrap hdg/1(<+/-pi) -> Saturation/1
  Sum3/1 -> dT/1
  Gain1/1 -> Sum3/2
  Gain5/1 -> Sum3/3
  Derivative1/1 -> Gain5/1

== system Aircraft6dof/Controller/Decoupled ==
  W_des : Inport
  W_tru : Inport  Port=2
  Q_tru : Inport  Port=3
  Tha_tru : Inport  Port=4
  Tha_des : Inport  Port=5
  U_tru : Inport  Port=6
  U_des : Inport  Port=7
  Constant : Constant  Value=K_decouple
  Constant1 : Constant  Value=0
  Constant2 : Constant  Value=0
  Demux : Demux  Outputs=2
  Gain : Gain  Gain=-1
  Mux : Mux
  Product : Product  Multiplication=Matrix(*)
  Scope : Scope
  Scope1 : Scope
  Sum : Sum  Inputs=|+-
  Sum1 : Sum  Inputs=-+|
  Sum2 : Sum  Inputs=|+-
  dAil : Outport  VectorParamsAs1DForOutWhenUnconnected=off
  dFlap : Outport  Port=2  VectorParamsAs1DForOutWhenUnconnected=off
  dElev : Outport  Port=3  VectorParamsAs1DForOutWhenUnconnected=off
  dRud : Outport  Port=4  VectorParamsAs1DForOutWhenUnconnected=off
  wires:
  Sum1/1 -> Mux/1
  W_des/1 -> Scope/1, Sum1/1
  Sum/1 -> Mux/4
  U_des/1 -> Sum/2
  Product/1 -> Demux/1
  Constant2/1 -> dRud/1
  Demux/2 -> dElev/1
  Demux/1 -> dFlap/1
  Constant1/1 -> dAil/1
  Constant/1 -> Gain/1
  Mux/1 -> Product/2
  U_tru/1 -> Sum/1
  Tha_tru/1 -> Sum2/1
  Q_tru/1 -> Mux/2
  W_tru/1 -> Scope1/1, Sum1/2
  Sum2/1 -> Mux/3
  Tha_des/1 -> Sum2/2
  Gain/1 -> Product/1

== system Aircraft6dof/Controller/Functional To Actual Control Allocation Mixing ==
  dA : Inport
  dF : Inport  Port=2
  dE : Inport  Port=3
  dR : Inport  Port=4
  Constant1 : Constant  Value=MixMatrix
  Demux : Demux
  Mux : Mux
  Product1 : Product  Multiplication=Matrix(*)
  dER : Outport  VectorParamsAs1DForOutWhenUnconnected=off
  dEL : Outport  Port=2  VectorParamsAs1DForOutWhenUnconnected=off
  dElev : Outport  Port=3  VectorParamsAs1DForOutWhenUnconnected=off
  dRud : Outport  Port=4  VectorParamsAs1DForOutWhenUnconnected=off
  wires:
  dA/1 -> Mux/1
  dF/1 -> Mux/2
  dE/1 -> Mux/3
  dR/1 -> Mux/4
  Demux/2 -> dEL/1
  Constant1/1 -> Product1/1
  Mux/1 -> Product1/2
  Demux/1 -> dER/1
  Demux/4 -> dRud/1
  Demux/3 -> dElev/1
  Product1/1 -> Demux/1

== system Aircraft6dof/Controller/LQG ==
  Vinf_des : Inport
  Vinf_meas : Inport  Port=2
  P_meas : Inport  Port=3
  Q_meas : Inport  Port=4
  R_meas : Inport  Port=5
  ax_meas : Inport  Port=6
  ay_meas : Inport  Port=7
  az_meas : Inport  Port=8
  hdg_meas : Inport  Port=9
  hdg_des : Inport  Port=10
  az_des : Inport  Port=11
  ax_des : Inport  Port=12
  Constant : Constant  Commented=on  Value=K_lqr
  Demux : Demux
  Mux : Mux  Inputs=8
  Product : Product  Commented=on  Multiplication=Matrix(*)
  Saturation : Saturate  UpperLimit=0.3  LowerLimit=-0.3
  State-Space : StateSpace  A=reg_lqg.a  B=reg_lqg.b  C=reg_lqg.c  D=reg_lqg.d  InitialCondition=0
  Sum : Sum  Inputs=|+-
  Sum1 : Sum  Inputs=-+|
  Sum2 : Sum  Inputs=|+-
  Sum3 : Sum  Inputs=|+-
  wrap hdg : Subsystem
  dAil : Outport  VectorParamsAs1DForOutWhenUnconnected=off
  dFlap : Outport  Port=2  VectorParamsAs1DForOutWhenUnconnected=off
  dElev : Outport  Port=3  VectorParamsAs1DForOutWhenUnconnected=off
  dRud : Outport  Port=4  VectorParamsAs1DForOutWhenUnconnected=off
  wires:
  Vinf_meas/1 -> Sum1/2
  P_meas/1 -> Mux/2
  Q_meas/1 -> Mux/3
  R_meas/1 -> Mux/4
  ax_meas/1 -> Sum3/1
  ay_meas/1 -> Mux/6
  az_meas/1 -> Sum2/1
  hdg_meas/1 -> Sum/1
  Mux/1 -> Product/2, State-Space/1
  Constant/1 -> Product/1
  Product/1 -> ?
  Demux/1 -> dAil/1
  Demux/2 -> dFlap/1
  Demux/3 -> dElev/1
  Demux/4 -> dRud/1
  State-Space/1 -> Demux/1
  hdg_des/1 -> Sum/2
  Sum/1 -> wrap hdg/1(hdg_err)
  Vinf_des/1 -> Sum1/1
  Sum1/1 -> Mux/1
  az_des/1 -> Sum2/2
  Sum2/1 -> Mux/7
  ax_des/1 -> Sum3/2
  Sum3/1 -> Mux/5
  wrap hdg/1(<+/-pi) -> Saturation/1
  Saturation/1 -> Mux/8

== system Aircraft6dof/Controller/No Feedback Open Loop Commands Steps, Ramps, Sweeps, etc ==
  Vinf_des : Inport
  hdg_des : Inport  Port=2
  Vinf_meas : Inport  Port=3
  hadg_meas : Inport  Port=4
  Clock : Clock  Commented=on
  Clock1 : Clock
  Elevator LookUP : Lookup_n-D  Commented=on  NumberOfTableDimensions=1  BreakpointsForDimension1=time_vector_elevator  Table=elevator_vector  InternalRulePriority=Speed  RndMeth=Simplest
  Rudder LookUP : Lookup_n-D  NumberOfTableDimensions=1  BreakpointsForDimension1=time_vector_rudder  Table=rudder_vector  InternalRulePriority=Speed  RndMeth=Simplest
  Terminator{,1,7,11} (4 alike) : Terminator
  dAil_cmd_rad : Constant  Value=0
  dElev_cmd_rad : Constant  Value=0
  dFlap_cmd_rad : Constant  Value=0
  dRud_cmd_rad : Constant  Commented=on  Value=0
  dAil : Outport  VectorParamsAs1DForOutWhenUnconnected=off
  dFlap : Outport  Port=2  VectorParamsAs1DForOutWhenUnconnected=off
  dElev : Outport  Port=3  VectorParamsAs1DForOutWhenUnconnected=off
  dRud : Outport  Port=4  VectorParamsAs1DForOutWhenUnconnected=off
  wires:
  dElev_cmd_rad/1 -> dElev/1
  Rudder LookUP/1 -> dRud/1
  dAil_cmd_rad/1 -> dAil/1
  Vinf_meas/1 -> Terminator/1
  hadg_meas/1 -> Terminator7/1
  hdg_des/1 -> Terminator11/1
  Clock/1 -> Elevator LookUP/1
  Clock1/1 -> Rudder LookUP/1
  dFlap_cmd_rad/1 -> dFlap/1
  Vinf_des/1 -> Terminator1/1

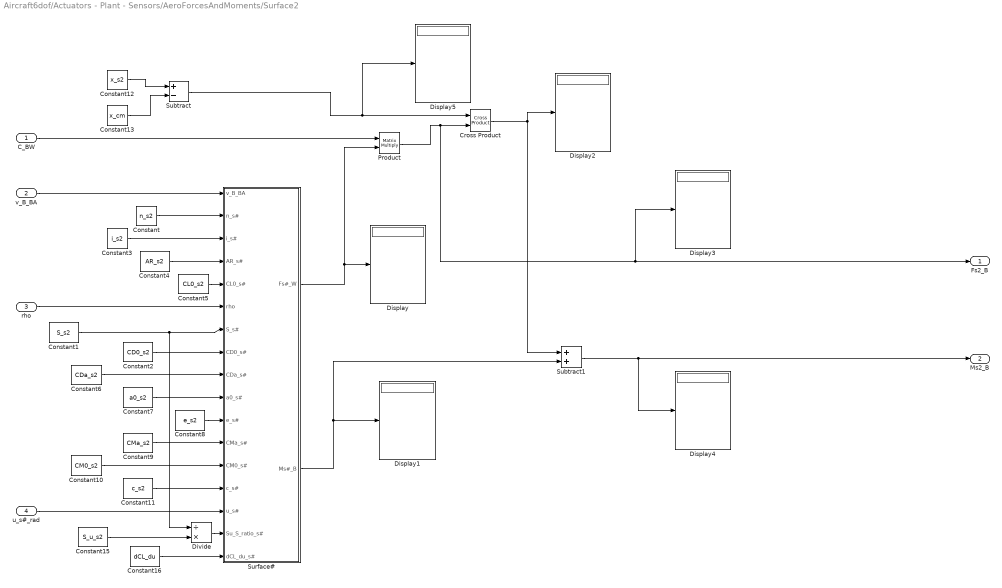
== system Aircraft6dof/Actuators - Plant - Sensors/AeroForcesAndMoments/Surface2 ==
  C_BW : Inport
  v_B_BA : Inport  Port=2
  rho : Inport  Port=3
  u_s#_rad : Inport  Port=4
  Constant : Constant  Value=n_s2
  Constant1 : Constant  Value=S_s2
  Constant10 : Constant  Value=CM0_s2
  Constant11 : Constant  Value=c_s2
  Constant12 : Constant  Value=x_s2
  Constant13 : Constant  Value=x_cm
  Constant15 : Constant  Value=S_u_s2
  Constant16 : Constant  Value=dCL_du
  Constant2 : Constant  Value=CD0_s2
  Constant3 : Constant  Value=i_s2
  Constant4 : Constant  Value=AR_s2
  Constant5 : Constant  Value=CL0_s2
  Constant6 : Constant  Value=CDa_s2
  Constant7 : Constant  Value=a0_s2
  Constant8 : Constant  Value=e_s2
  Constant9 : Constant  Value=CMa_s2
  Cross Product : vrlib/Utilities/Cross Product
  Display{,1..5} (6 alike) : Display
  Divide : Product  Inputs=/*
  Product : Product  Multiplication=Matrix(*)
  Subtract : Sum  Inputs=+-
  Subtract1 : Sum
  Surface# : Subsystem
  Fs2_B : Outport  VectorParamsAs1DForOutWhenUnconnected=off
  Ms2_B : Outport  Port=2  VectorParamsAs1DForOutWhenUnconnected=off
  wires:
  Subtract/1 -> Display5/1, Cross Product/1
  C_BW/1 -> Product/1
  Constant12/1 -> Subtract/1
  Constant13/1 -> Subtract/2
  Cross Product/1 -> Subtract1/1, Display2/1
  Product/1 -> Fs2_B/1, Display3/1, Cross Product/2
  Subtract1/1 -> Ms2_B/1, Display4/1
  Surface#/2(Ms#_B) -> Subtract1/2, Display1/1
  Constant10/1 -> Surface#/13(CM0_s#)
  Surface#/1(Fs#_W) -> Product/2, Display/1
  Constant11/1 -> Surface#/14(c_s#)
  Constant9/1 -> Surface#/12(CMa_s#)
  Constant7/1 -> Surface#/10(a0_s#)
  v_B_BA/1 -> Surface#/1(v_B_BA)
  Constant/1 -> Surface#/2(n_s#)
  Constant3/1 -> Surface#/3(i_s#)
  Constant4/1 -> Surface#/4(AR_s#)
  Constant5/1 -> Surface#/5(CL0_s#)
  rho/1 -> Surface#/6(rho)
  Constant2/1 -> Surface#/8(CD0_s#)
  Constant6/1 -> Surface#/9(CDa_s#)
  Constant8/1 -> Surface#/11(e_s#)
  Constant1/1 -> Divide/1, Surface#/7(S_s#)
  u_s#_rad/1 -> Surface#/15(u_s#)
  Constant15/1 -> Divide/2
  Constant16/1 -> Surface#/17(dCL_du_s#)
  Divide/1 -> Surface#/16(Su_S_ratio_s#)

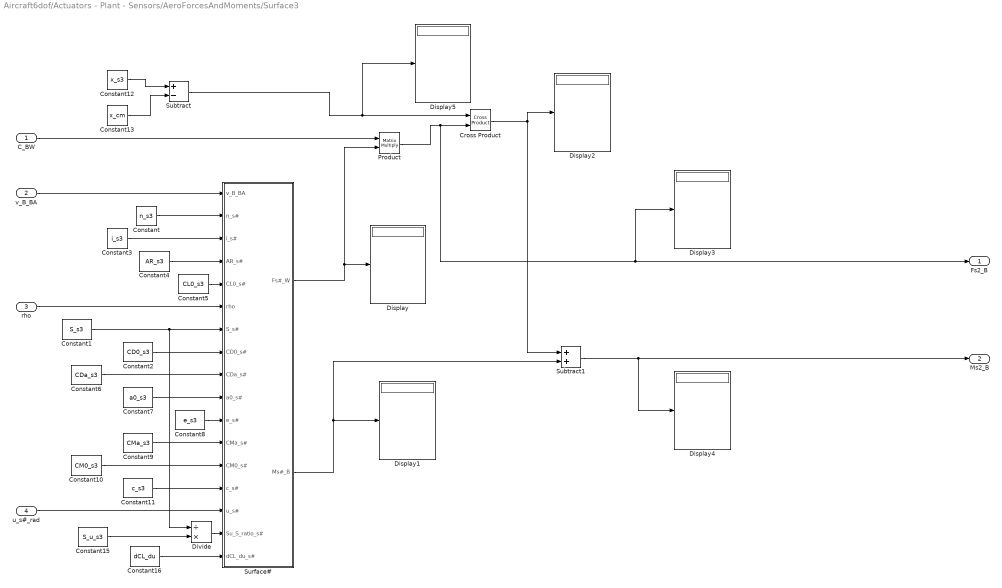
== system Aircraft6dof/Actuators - Plant - Sensors/AeroForcesAndMoments/Surface3 ==
  C_BW : Inport
  v_B_BA : Inport  Port=2
  rho : Inport  Port=3
  u_s#_rad : Inport  Port=4
  Constant : Constant  Value=n_s3
  Constant1 : Constant  Value=S_s3
  Constant10 : Constant  Value=CM0_s3
  Constant11 : Constant  Value=c_s3
  Constant12 : Constant  Value=x_s3
  Constant13 : Constant  Value=x_cm
  Constant15 : Constant  Value=S_u_s3
  Constant16 : Constant  Value=dCL_du
  Constant2 : Constant  Value=CD0_s3
  Constant3 : Constant  Value=i_s3
  Constant4 : Constant  Value=AR_s3
  Constant5 : Constant  Value=CL0_s3
  Constant6 : Constant  Value=CDa_s3
  Constant7 : Constant  Value=a0_s3
  Constant8 : Constant  Value=e_s3
  Constant9 : Constant  Value=CMa_s3
  Cross Product : vrlib/Utilities/Cross Product
  Display{,1..5} (6 alike) : Display
  Divide : Product  Inputs=/*
  Product : Product  Multiplication=Matrix(*)
  Subtract : Sum  Inputs=+-
  Subtract1 : Sum
  Surface# : Subsystem
  Fs2_B : Outport  VectorParamsAs1DForOutWhenUnconnected=off
  Ms2_B : Outport  Port=2  VectorParamsAs1DForOutWhenUnconnected=off
  wires:
  Subtract/1 -> Display5/1, Cross Product/1
  C_BW/1 -> Product/1
  Constant12/1 -> Subtract/1
  Constant13/1 -> Subtract/2
  Cross Product/1 -> Subtract1/1, Display2/1
  Product/1 -> Fs2_B/1, Display3/1, Cross Product/2
  Subtract1/1 -> Ms2_B/1, Display4/1
  Surface#/2(Ms#_B) -> Subtract1/2, Display1/1
  Constant10/1 -> Surface#/13(CM0_s#)
  Surface#/1(Fs#_W) -> Product/2, Display/1
  Constant11/1 -> Surface#/14(c_s#)
  Constant9/1 -> Surface#/12(CMa_s#)
  Constant7/1 -> Surface#/10(a0_s#)
  v_B_BA/1 -> Surface#/1(v_B_BA)
  Constant/1 -> Surface#/2(n_s#)
  Constant3/1 -> Surface#/3(i_s#)
  Constant4/1 -> Surface#/4(AR_s#)
  Constant5/1 -> Surface#/5(CL0_s#)
  rho/1 -> Surface#/6(rho)
  Constant2/1 -> Surface#/8(CD0_s#)
  Constant6/1 -> Surface#/9(CDa_s#)
  Constant8/1 -> Surface#/11(e_s#)
  Constant1/1 -> Divide/1, Surface#/7(S_s#)
  u_s#_rad/1 -> Surface#/15(u_s#)
  Constant15/1 -> Divide/2
  Constant16/1 -> Surface#/17(dCL_du_s#)
  Divide/1 -> Surface#/16(Su_S_ratio_s#)

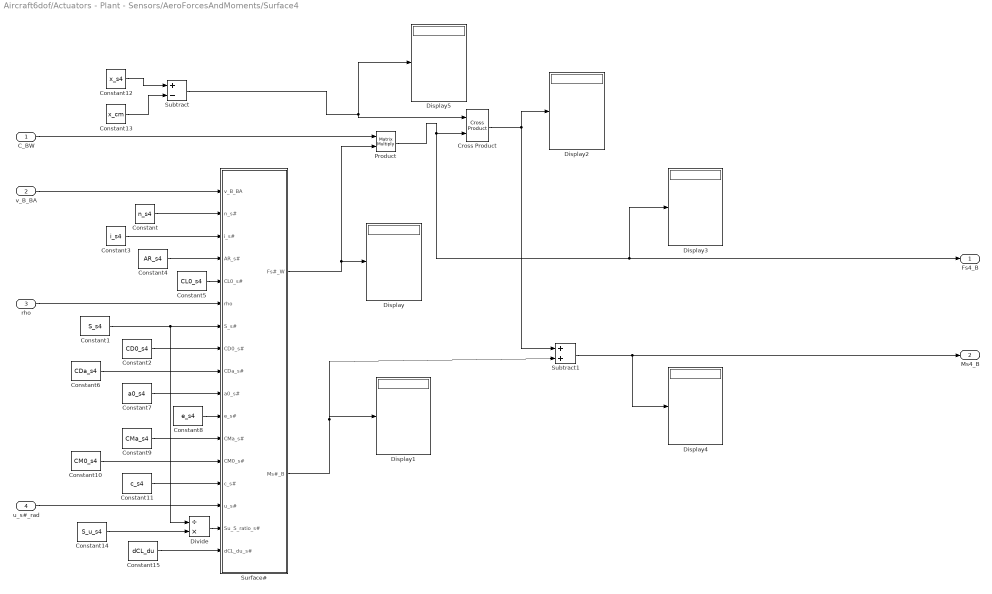
== system Aircraft6dof/Actuators - Plant - Sensors/AeroForcesAndMoments/Surface4 ==
  C_BW : Inport
  v_B_BA : Inport  Port=2
  rho : Inport  Port=3
  u_s#_rad : Inport  Port=4
  Constant : Constant  Value=n_s4
  Constant1 : Constant  Value=S_s4
  Constant10 : Constant  Value=CM0_s4
  Constant11 : Constant  Value=c_s4
  Constant12 : Constant  Value=x_s4
  Constant13 : Constant  Value=x_cm
  Constant14 : Constant  Value=S_u_s4
  Constant15 : Constant  Value=dCL_du
  Constant2 : Constant  Value=CD0_s4
  Constant3 : Constant  Value=i_s4
  Constant4 : Constant  Value=AR_s4
  Constant5 : Constant  Value=CL0_s4
  Constant6 : Constant  Value=CDa_s4
  Constant7 : Constant  Value=a0_s4
  Constant8 : Constant  Value=e_s4
  Constant9 : Constant  Value=CMa_s4
  Cross Product : vrlib/Utilities/Cross Product
  Display{,1..5} (6 alike) : Display
  Divide : Product  Inputs=/*
  Product : Product  Multiplication=Matrix(*)
  Subtract : Sum  Inputs=+-
  Subtract1 : Sum
  Surface# : Subsystem
  Fs4_B : Outport  VectorParamsAs1DForOutWhenUnconnected=off
  Ms4_B : Outport  Port=2  VectorParamsAs1DForOutWhenUnconnected=off
  wires:
  Subtract/1 -> Display5/1, Cross Product/1
  C_BW/1 -> Product/1
  Constant12/1 -> Subtract/1
  Constant13/1 -> Subtract/2
  Cross Product/1 -> Display2/1, Subtract1/1
  Product/1 -> Fs4_B/1, Display3/1, Cross Product/2
  Subtract1/1 -> Ms4_B/1, Display4/1
  Surface#/2(Ms#_B) -> Subtract1/2, Display1/1
  Constant10/1 -> Surface#/13(CM0_s#)
  Surface#/1(Fs#_W) -> Product/2, Display/1
  Constant11/1 -> Surface#/14(c_s#)
  Constant9/1 -> Surface#/12(CMa_s#)
  Constant7/1 -> Surface#/10(a0_s#)
  v_B_BA/1 -> Surface#/1(v_B_BA)
  Constant/1 -> Surface#/2(n_s#)
  Constant3/1 -> Surface#/3(i_s#)
  Constant4/1 -> Surface#/4(AR_s#)
  Constant5/1 -> Surface#/5(CL0_s#)
  rho/1 -> Surface#/6(rho)
  Constant1/1 -> Divide/1, Surface#/7(S_s#)
  Constant2/1 -> Surface#/8(CD0_s#)
  Constant6/1 -> Surface#/9(CDa_s#)
  Constant8/1 -> Surface#/11(e_s#)
  u_s#_rad/1 -> Surface#/15(u_s#)
  Divide/1 -> Surface#/16(Su_S_ratio_s#)
  Constant14/1 -> Divide/2
  Constant15/1 -> Surface#/17(dCL_du_s#)

== system Aircraft6dof/Actuators - Plant - Sensors/AeroForcesAndMoments/Surface5 ==
  C_BW : Inport
  v_B_BA : Inport  Port=2
  rho : Inport  Port=3
  u_s#_rad : Inport  Port=4
  Constant : Constant  Value=n_s5
  Constant1 : Constant  Value=S_s5
  Constant10 : Constant  Value=CM0_s5
  Constant11 : Constant  Value=c_s5
  Constant12 : Constant  Value=x_s5
  Constant13 : Constant  Value=x_cm
  Constant15 : Constant  Value=S_u_s5
  Constant16 : Constant  Value=dCL_du
  Constant2 : Constant  Value=CD0_s5
  Constant3 : Constant  Value=i_s5
  Constant4 : Constant  Value=AR_s5
  Constant5 : Constant  Value=CL0_s5
  Constant6 : Constant  Value=CDa_s5
  Constant7 : Constant  Value=a0_s5
  Constant8 : Constant  Value=e_s5
  Constant9 : Constant  Value=CMa_s5
  Cross Product : vrlib/Utilities/Cross Product
  Display{,1..5} (6 alike) : Display
  Divide : Product  Inputs=/*
  Product : Product  Multiplication=Matrix(*)
  Subtract : Sum  Inputs=+-
  Subtract1 : Sum
  Surface# : Subsystem
  Fs5_B : Outport  VectorParamsAs1DForOutWhenUnconnected=off
  Ms5_B : Outport  Port=2  VectorParamsAs1DForOutWhenUnconnected=off
  wires:
  Constant8/1 -> Surface#/11(e_s#)
  Constant6/1 -> Surface#/9(CDa_s#)
  Constant2/1 -> Surface#/8(CD0_s#)
  rho/1 -> Surface#/6(rho)
  Constant5/1 -> Surface#/5(CL0_s#)
  Constant4/1 -> Surface#/4(AR_s#)
  Constant3/1 -> Surface#/3(i_s#)
  Constant/1 -> Surface#/2(n_s#)
  v_B_BA/1 -> Surface#/1(v_B_BA)
  Constant7/1 -> Surface#/10(a0_s#)
  Constant9/1 -> Surface#/12(CMa_s#)
  Constant11/1 -> Surface#/14(c_s#)
  Surface#/1(Fs#_W) -> Display/1, Product/2
  Constant10/1 -> Surface#/13(CM0_s#)
  Surface#/2(Ms#_B) -> Display1/1, Subtract1/2
  Subtract1/1 -> Display4/1, Ms5_B/1
  Product/1 -> Cross Product/2, Display3/1, Fs5_B/1
  Cross Product/1 -> Display2/1, Subtract1/1
  Constant13/1 -> Subtract/2
  Constant12/1 -> Subtract/1
  C_BW/1 -> Product/1
  Subtract/1 -> Cross Product/1, Display5/1
  Constant1/1 -> Surface#/7(S_s#), Divide/1
  u_s#_rad/1 -> Surface#/15(u_s#)
  Constant15/1 -> Divide/2
  Constant16/1 -> Surface#/17(dCL_du_s#)
  Divide/1 -> Surface#/16(Su_S_ratio_s#)

== system Aircraft6dof/Actuators - Plant - Sensors/Equations Of Motion State Equations/Earth Model ==
  p_E_E_BE : Inport
  Constant1 : Constant  Value=Rearth
  Constant6 : Constant  Value=g_E_N
  Terminator : Terminator
  Rearth : Outport  VectorParamsAs1DForOutWhenUnconnected=off
  g_N : Outport  Port=2  VectorParamsAs1DForOutWhenUnconnected=off
  wires:
  Constant6/1 -> g_N/1
  p_E_E_BE/1 -> Terminator/1
  Constant1/1 -> Rearth/1

== system Aircraft6dof/Actuators - Plant - Sensors/Equations Of Motion State Equations/QUAT2ATT ==
  q : Inport
  Mux : Mux  Inputs=3
  Trigonometric Function1 : Trigonometry  Operator=atan2
  Trigonometric Function3 : Trigonometry  Operator=atan2
  fcn1 : Fcn  Expr=2*(u[2]*u[3] + u[1]*u[4])
  fcn2 : Fcn  Expr=u[1]*u[1] + u[2]*u[2] - u[3]*u[3] - u[4]*u[4]
  fcn3 : Fcn  Expr=-2*(u[2]*u[4] - u[1]*u[3])
  fcn4 : Fcn  Expr=2*(u[3]*u[4] + u[1]*u[2])
  fcn5 : Fcn  Expr=u[1]*u[1] - u[2]*u[2] - u[3]*u[3] + u[4]*u[4]
  trigFcn : Trigonometry  Operator=asin
  ATT : Outport  VectorParamsAs1DForOutWhenUnconnected=off
  wires:
  q/1 -> fcn2/1, fcn1/1, fcn4/1, fcn5/1, fcn3/1
  Trigonometric Function3/1 -> Mux/1  "psi"
  trigFcn/1 -> Mux/2  "theta"
  Trigonometric Function1/1 -> Mux/3  "phi"
  Mux/1 -> ATT/1
  fcn3/1 -> trigFcn/1
  fcn1/1 -> Trigonometric Function1/1
  fcn2/1 -> Trigonometric Function1/2
  fcn4/1 -> Trigonometric Function3/1
  fcn5/1 -> Trigonometric Function3/2
